simulink model "xb_pfb_fir_16k_4tap_core"  (Simulink 7.8)
settings: Solver=ode45  StartTime=0.0  StopTime=10.0  RelTol=1e-3
libraries: xbsIndex_r4 x287, casper_library_misc x8
(part 3 of 9)

== system xb_pfb_fir_16k_4tap_core/pfb_fir1/pfb_row_11/ri_to_c0 ==
  re : Inport
  im : Inport  Port=2
  concat : xbsIndex_r4/Concat  num_inputs=2  dbl_ovrd=off  block_type=concat
  force_im : xbsIndex_r4/Reinterpret  force_arith_type=on  arith_type=Unsigned  force_bin_pt=on  bin_pt=0  block_type=reinterpret
  force_re : xbsIndex_r4/Reinterpret  force_arith_type=on  arith_type=Unsigned  force_bin_pt=on  bin_pt=0  block_type=reinterpret
  c : Outport
  wires:
  force_re/1 -> concat/1
  re/1 -> force_re/1
  force_im/1 -> concat/2
  im/1 -> force_im/1
  concat/1 -> c/1

== system xb_pfb_fir_16k_4tap_core/pfb_fir1/pfb_row_11/sync_delay ==
  In : Inport
  Constant : xbsIndex_r4/Constant  const=1  gui_display_data_type=Fixed-point  arith_type=Unsigned  n_bits=14  bin_pt=0  preci_type=Single  exp_width=8  frac_width=24  explicit_period=on  period=1  equ=P=C  opselect=C  inp2=PCIN>>17  opr=+  inp1=P  carry=CIN  dbl_ovrd=off  block_type=constant
  Constant1 : xbsIndex_r4/Constant  const=0  gui_display_data_type=Fixed-point  arith_type=Unsigned  n_bits=14  bin_pt=0  preci_type=Single  exp_width=8  frac_width=24  explicit_period=on  period=1  equ=P=C  opselect=C  inp2=PCIN>>17  opr=+  inp1=P  carry=CIN  dbl_ovrd=off  block_type=constant
  Constant2 : xbsIndex_r4/Constant  const=12291  gui_display_data_type=Fixed-point  arith_type=Unsigned  n_bits=14  bin_pt=0  preci_type=Single  exp_width=8  frac_width=24  explicit_period=on  period=1  equ=P=C  opselect=C  inp2=PCIN>>17  opr=+  inp1=P  carry=CIN  dbl_ovrd=off  block_type=constant
  Counter : xbsIndex_r4/Counter  cnt_type=Free Running  cnt_to=Inf  operation=Down  start_count=0  cnt_by_val=1  arith_type=Unsigned  n_bits=14  bin_pt=0  load_pin=on  rst=off  en=on  explicit_period=on  period=1  dbl_ovrd=off  use_behavioral_HDL=off  implementation=Fabric  use_rpm=on  block_type=counter
  Logical : xbsIndex_r4/Logical  logical_function=OR  inputs=2  en=off  latency=0  precision=Full  arith_type=Unsigned  n_bits=8  bin_pt=2  align_bp=on  dbl_ovrd=off  block_type=logical
  Relational : xbsIndex_r4/Relational  mode=a=b  en=off  latency=0  dbl_ovrd=off  block_type=relational
  Relational1 : xbsIndex_r4/Relational  mode=a!=b  en=off  latency=0  dbl_ovrd=off  block_type=relational
  Out : Outport
  wires:
  In/1 -> Logical/1, Counter/1
  Counter/1 -> Relational1/1, Relational/2
  Relational1/1 -> Logical/2
  Constant1/1 -> Relational1/2
  Relational/1 -> Out/1
  Constant/1 -> Relational/1
  Logical/1 -> Counter/3
  Constant2/1 -> Counter/2

== system xb_pfb_fir_16k_4tap_core/pfb_fir1/pfb_row_11/tap_split_1 ==
  inport : Inport
  Reinterp1 : xbsIndex_r4/Reinterpret  force_arith_type=on  arith_type="Signed  (2's comp)"  force_bin_pt=on  bin_pt=7  block_type=reinterpret
  Reinterp2 : xbsIndex_r4/Reinterpret  force_arith_type=on  arith_type="Signed  (2's comp)"  force_bin_pt=on  bin_pt=7  block_type=reinterpret
  Slice1 : xbsIndex_r4/Slice  nbits=8  boolean_output=off  mode=Upper Bit Location + Width  bit1=-0  base1=MSB of Input  bit0=0  base0=LSB of Input  dbl_ovrd=off  block_type=slice
  Slice2 : xbsIndex_r4/Slice  nbits=8  boolean_output=off  mode=Upper Bit Location + Width  bit1=-8  base1=MSB of Input  bit0=0  base0=LSB of Input  dbl_ovrd=off  block_type=slice
  outport1 : Outport
  outport2 : Outport  Port=2
  wires:
  inport/1 -> Slice2/1, Slice1/1
  Reinterp2/1 -> outport2/1
  Slice2/1 -> Reinterp2/1  "slice_out2"
  Reinterp1/1 -> outport1/1
  Slice1/1 -> Reinterp1/1  "slice_out1"

== system xb_pfb_fir_16k_4tap_core/pfb_fir1/pfb_row_11/tap_split_2 ==
  inport : Inport
  Reinterp1 : xbsIndex_r4/Reinterpret  force_arith_type=on  arith_type="Signed  (2's comp)"  force_bin_pt=on  bin_pt=7  block_type=reinterpret
  Reinterp2 : xbsIndex_r4/Reinterpret  force_arith_type=on  arith_type="Signed  (2's comp)"  force_bin_pt=on  bin_pt=7  block_type=reinterpret
  Slice1 : xbsIndex_r4/Slice  nbits=8  boolean_output=off  mode=Upper Bit Location + Width  bit1=-0  base1=MSB of Input  bit0=0  base0=LSB of Input  dbl_ovrd=off  block_type=slice
  Slice2 : xbsIndex_r4/Slice  nbits=8  boolean_output=off  mode=Upper Bit Location + Width  bit1=-8  base1=MSB of Input  bit0=0  base0=LSB of Input  dbl_ovrd=off  block_type=slice
  outport1 : Outport
  outport2 : Outport  Port=2
  wires:
  inport/1 -> Slice2/1, Slice1/1
  Reinterp2/1 -> outport2/1
  Slice2/1 -> Reinterp2/1  "slice_out2"
  Reinterp1/1 -> outport1/1
  Slice1/1 -> Reinterp1/1  "slice_out1"

== system xb_pfb_fir_16k_4tap_core/pfb_fir1/pfb_row_11/tap_split_3 ==
  inport : Inport
  Reinterp1 : xbsIndex_r4/Reinterpret  force_arith_type=on  arith_type="Signed  (2's comp)"  force_bin_pt=on  bin_pt=7  block_type=reinterpret
  Reinterp2 : xbsIndex_r4/Reinterpret  force_arith_type=on  arith_type="Signed  (2's comp)"  force_bin_pt=on  bin_pt=7  block_type=reinterpret
  Slice1 : xbsIndex_r4/Slice  nbits=8  boolean_output=off  mode=Upper Bit Location + Width  bit1=-0  base1=MSB of Input  bit0=0  base0=LSB of Input  dbl_ovrd=off  block_type=slice
  Slice2 : xbsIndex_r4/Slice  nbits=8  boolean_output=off  mode=Upper Bit Location + Width  bit1=-8  base1=MSB of Input  bit0=0  base0=LSB of Input  dbl_ovrd=off  block_type=slice
  outport1 : Outport
  outport2 : Outport  Port=2
  wires:
  inport/1 -> Slice2/1, Slice1/1
  Reinterp2/1 -> outport2/1
  Slice2/1 -> Reinterp2/1  "slice_out2"
  Reinterp1/1 -> outport1/1
  Slice1/1 -> Reinterp1/1  "slice_out1"

== system xb_pfb_fir_16k_4tap_core/pfb_fir1/pfb_row_11/tap_split_4 ==
  inport : Inport
  Reinterp1 : xbsIndex_r4/Reinterpret  force_arith_type=on  arith_type="Signed  (2's comp)"  force_bin_pt=on  bin_pt=7  block_type=reinterpret
  Reinterp2 : xbsIndex_r4/Reinterpret  force_arith_type=on  arith_type="Signed  (2's comp)"  force_bin_pt=on  bin_pt=7  block_type=reinterpret
  Slice1 : xbsIndex_r4/Slice  nbits=8  boolean_output=off  mode=Upper Bit Location + Width  bit1=-0  base1=MSB of Input  bit0=0  base0=LSB of Input  dbl_ovrd=off  block_type=slice
  Slice2 : xbsIndex_r4/Slice  nbits=8  boolean_output=off  mode=Upper Bit Location + Width  bit1=-8  base1=MSB of Input  bit0=0  base0=LSB of Input  dbl_ovrd=off  block_type=slice
  outport1 : Outport
  outport2 : Outport  Port=2
  wires:
  inport/1 -> Slice2/1, Slice1/1
  Reinterp2/1 -> outport2/1
  Slice2/1 -> Reinterp2/1  "slice_out2"
  Reinterp1/1 -> outport1/1
  Slice1/1 -> Reinterp1/1  "slice_out1"

== system xb_pfb_fir_16k_4tap_core/pfb_fir1/pfb_row_12/adder_tree1 ==
  sync : Inport
  din_1 : Inport  Port=2
  din_2 : Inport  Port=3
  din_3 : Inport  Port=4
  din_4 : Inport  Port=5
  adder_0 : xbsIndex_r4/AddSub  mode=Addition  use_carryin=off  use_carryout=off  en=off  latency=2  precision=Full  arith_type=Unsigned  n_bits=18  bin_pt=17  quantization="Round  (unbiased: +/- Inf)"  overflow=Wrap  dbl_ovrd=off  use_behavioral_HDL=on  hw_selection=Fabric  pipelined=off  block_type=addsub
  adder_1 : xbsIndex_r4/AddSub  mode=Addition  use_carryin=off  use_carryout=off  en=off  latency=2  precision=Full  arith_type=Unsigned  n_bits=18  bin_pt=17  quantization="Round  (unbiased: +/- Inf)"  overflow=Wrap  dbl_ovrd=off  use_behavioral_HDL=on  hw_selection=Fabric  pipelined=off  block_type=addsub
  adder_2 : xbsIndex_r4/AddSub  mode=Addition  use_carryin=off  use_carryout=off  en=off  latency=2  precision=Full  arith_type=Unsigned  n_bits=18  bin_pt=17  quantization="Round  (unbiased: +/- Inf)"  overflow=Wrap  dbl_ovrd=off  use_behavioral_HDL=on  hw_selection=Fabric  pipelined=off  block_type=addsub
  sync_delay : xbsIndex_r4/Delay  rst=off  infoeditControl=Selection of Reset will increase slice count due to use of real FFs and instead of SRLs  en=off  latency=4  dbl_ovrd=off  reg_retiming=off  block_type=delay
  sync_out : Outport
  dout : Outport  Port=2
  wires:
  adder_2/1 -> dout/1
  adder_0/1 -> adder_2/2
  adder_1/1 -> adder_2/1
  din_3/1 -> adder_1/2
  din_4/1 -> adder_1/1
  din_1/1 -> adder_0/2
  din_2/1 -> adder_0/1
  sync_delay/1 -> sync_out/1
  sync/1 -> sync_delay/1

== system xb_pfb_fir_16k_4tap_core/pfb_fir1/pfb_row_12/adder_tree2 ==
  sync : Inport
  din_1 : Inport  Port=2
  din_2 : Inport  Port=3
  din_3 : Inport  Port=4
  din_4 : Inport  Port=5
  adder_0 : xbsIndex_r4/AddSub  mode=Addition  use_carryin=off  use_carryout=off  en=off  latency=2  precision=Full  arith_type=Unsigned  n_bits=18  bin_pt=17  quantization="Round  (unbiased: +/- Inf)"  overflow=Wrap  dbl_ovrd=off  use_behavioral_HDL=on  hw_selection=Fabric  pipelined=off  block_type=addsub
  adder_1 : xbsIndex_r4/AddSub  mode=Addition  use_carryin=off  use_carryout=off  en=off  latency=2  precision=Full  arith_type=Unsigned  n_bits=18  bin_pt=17  quantization="Round  (unbiased: +/- Inf)"  overflow=Wrap  dbl_ovrd=off  use_behavioral_HDL=on  hw_selection=Fabric  pipelined=off  block_type=addsub
  adder_2 : xbsIndex_r4/AddSub  mode=Addition  use_carryin=off  use_carryout=off  en=off  latency=2  precision=Full  arith_type=Unsigned  n_bits=18  bin_pt=17  quantization="Round  (unbiased: +/- Inf)"  overflow=Wrap  dbl_ovrd=off  use_behavioral_HDL=on  hw_selection=Fabric  pipelined=off  block_type=addsub
  sync_delay : xbsIndex_r4/Delay  rst=off  infoeditControl=Selection of Reset will increase slice count due to use of real FFs and instead of SRLs  en=off  latency=4  dbl_ovrd=off  reg_retiming=off  block_type=delay
  sync_out : Outport
  dout : Outport  Port=2
  wires:
  adder_2/1 -> dout/1
  adder_0/1 -> adder_2/2
  adder_1/1 -> adder_2/1
  din_3/1 -> adder_1/2
  din_4/1 -> adder_1/1
  din_1/1 -> adder_0/2
  din_2/1 -> adder_0/1
  sync_delay/1 -> sync_out/1
  sync/1 -> sync_delay/1

== system xb_pfb_fir_16k_4tap_core/pfb_fir1/pfb_row_12/delay_bram2 ==
  din_1_1 : Inport
  Constant1 : xbsIndex_r4/Constant  const=0  gui_display_data_type=Fixed-point  arith_type=Unsigned  n_bits=2  bin_pt=0  preci_type=Single  exp_width=8  frac_width=24  explicit_period=on  period=1  equ=P=C  opselect=C  inp2=PCIN>>17  opr=+  inp1=P  carry=CIN  dbl_ovrd=off  block_type=constant
  Constant2 : xbsIndex_r4/Constant  const=1  gui_display_data_type=Fixed-point  arith_type=Boolean  n_bits=1  bin_pt=0  preci_type=Single  exp_width=8  frac_width=24  explicit_period=on  period=1  equ=P=C  opselect=C  inp2=PCIN>>17  opr=+  inp1=P  carry=CIN  dbl_ovrd=off  block_type=constant
  bram1 : xbsIndex_r4/Single Port RAM  depth=4  initVector=0  distributed_mem=Block RAM  write_mode=Read Before Write  rst=off  init_reg=0  en=off  latency=4  dbl_ovrd=off  optimize=Area  use_rpm=off  block_type=spram
  dout_1_1 : Outport
  wires:
  bram1/1 -> dout_1_1/1
  Constant2/1 -> bram1/3
  din_1_1/1 -> bram1/2
  Constant1/1 -> bram1/1

== system xb_pfb_fir_16k_4tap_core/pfb_fir1/pfb_row_12/delay_bram3 ==
  din_1_1 : Inport
  Constant1 : xbsIndex_r4/Constant  const=0  gui_display_data_type=Fixed-point  arith_type=Unsigned  n_bits=2  bin_pt=0  preci_type=Single  exp_width=8  frac_width=24  explicit_period=on  period=1  equ=P=C  opselect=C  inp2=PCIN>>17  opr=+  inp1=P  carry=CIN  dbl_ovrd=off  block_type=constant
  Constant2 : xbsIndex_r4/Constant  const=1  gui_display_data_type=Fixed-point  arith_type=Boolean  n_bits=1  bin_pt=0  preci_type=Single  exp_width=8  frac_width=24  explicit_period=on  period=1  equ=P=C  opselect=C  inp2=PCIN>>17  opr=+  inp1=P  carry=CIN  dbl_ovrd=off  block_type=constant
  bram1 : xbsIndex_r4/Single Port RAM  depth=4  initVector=0  distributed_mem=Block RAM  write_mode=Read Before Write  rst=off  init_reg=0  en=off  latency=4  dbl_ovrd=off  optimize=Area  use_rpm=off  block_type=spram
  dout_1_1 : Outport
  wires:
  bram1/1 -> dout_1_1/1
  Constant2/1 -> bram1/3
  din_1_1/1 -> bram1/2
  Constant1/1 -> bram1/1

== system xb_pfb_fir_16k_4tap_core/pfb_fir1/pfb_row_12/delay_bram4 ==
  din_1_1 : Inport
  Constant1 : xbsIndex_r4/Constant  const=0  gui_display_data_type=Fixed-point  arith_type=Signed (2's comp)  n_bits=2  bin_pt=0  preci_type=Single  exp_width=8  frac_width=24  explicit_period=on  period=1  equ=P=C  opselect=C  inp2=PCIN>>17  opr=+  inp1=P  carry=CIN  dbl_ovrd=off  block_type=constant
  Constant2 : xbsIndex_r4/Constant  const=1  gui_display_data_type=Fixed-point  arith_type=Boolean  n_bits=1  bin_pt=0  preci_type=Single  exp_width=8  frac_width=24  explicit_period=on  period=1  equ=P=C  opselect=C  inp2=PCIN>>17  opr=+  inp1=P  carry=CIN  dbl_ovrd=off  block_type=constant
  bram1 : xbsIndex_r4/Single Port RAM  depth=4  initVector=0  distributed_mem=Block RAM  write_mode=Read Before Write  rst=off  init_reg=0  en=off  latency=4  dbl_ovrd=off  optimize=Area  use_rpm=off  block_type=spram
  dout_1_1 : Outport
  wires:
  bram1/1 -> dout_1_1/1
  Constant2/1 -> bram1/3
  din_1_1/1 -> bram1/2
  Constant1/1 -> bram1/1

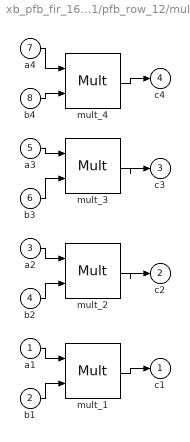
== system xb_pfb_fir_16k_4tap_core/pfb_fir1/pfb_row_12/mult1 ==
  a1 : Inport
  b1 : Inport  Port=2
  a2 : Inport  Port=3
  b2 : Inport  Port=4
  a3 : Inport  Port=5
  b3 : Inport  Port=6
  a4 : Inport  Port=7
  b4 : Inport  Port=8
  mult_{1..4} (4 alike) : xbsIndex_r4/Mult  precision=Full  arith_type="Signed  (2's comp)"  n_bits=16  bin_pt=14  quantization=Truncate  overflow=Wrap  en=off  latency=3  dbl_ovrd=off  use_behavioral_HDL=off  opt=Speed  use_embedded=on  optimum_pipeline=off  pipeline=on  use_rpm=on  placement_style=Triangular  block_type=mult
  c1 : Outport
  c2 : Outport  Port=2
  c3 : Outport  Port=3
  c4 : Outport  Port=4
  wires:
  mult_4/1 -> c4/1
  b4/1 -> mult_4/2
  a4/1 -> mult_4/1
  mult_3/1 -> c3/1
  b3/1 -> mult_3/2
  a3/1 -> mult_3/1
  mult_2/1 -> c2/1
  b2/1 -> mult_2/2
  a2/1 -> mult_2/1
  mult_1/1 -> c1/1
  b1/1 -> mult_1/2
  a1/1 -> mult_1/1

== system xb_pfb_fir_16k_4tap_core/pfb_fir1/pfb_row_12/mult2 ==
  a1 : Inport
  b1 : Inport  Port=2
  a2 : Inport  Port=3
  b2 : Inport  Port=4
  a3 : Inport  Port=5
  b3 : Inport  Port=6
  a4 : Inport  Port=7
  b4 : Inport  Port=8
  mult_{1..4} (4 alike) : xbsIndex_r4/Mult  precision=Full  arith_type="Signed  (2's comp)"  n_bits=16  bin_pt=14  quantization=Truncate  overflow=Wrap  en=off  latency=3  dbl_ovrd=off  use_behavioral_HDL=off  opt=Speed  use_embedded=on  optimum_pipeline=off  pipeline=on  use_rpm=on  placement_style=Triangular  block_type=mult
  c1 : Outport
  c2 : Outport  Port=2
  c3 : Outport  Port=3
  c4 : Outport  Port=4
  wires:
  mult_4/1 -> c4/1
  b4/1 -> mult_4/2
  a4/1 -> mult_4/1
  mult_3/1 -> c3/1
  b3/1 -> mult_3/2
  a3/1 -> mult_3/1
  mult_2/1 -> c2/1
  b2/1 -> mult_2/2
  a2/1 -> mult_2/1
  mult_1/1 -> c1/1
  b1/1 -> mult_1/2
  a1/1 -> mult_1/1
